simulink model "SWC_ETE_type"  (R2024a)
settings: Solver=FixedStepDiscrete  StartTime=0.0  StopTime=10.0  RelTol=1e-3
values from neighbouring files (symbols this model uses):
  C_FOC_SAMPLE_TIME = single(0.0001)    [vcu_local_hdr.m]
  ENUM_SENSORFOCMODE_CURRENTRDCTEMP = uint8(  2  )    [vcu_local_hdr.m]
  ENUM_SENSORFOCMODE_FAKERDC = uint8(  1  )    [vcu_local_hdr.m]
  ENUM_SENSORFOCMODE_RDCALIGN = uint8(  3  )    [vcu_local_hdr.m]
  ENUM_SENSORMODE_RDC = uint8(  0  )    [vcu_local_hdr.m]
  FALSE = boolean( 0 )    [vcu_local_hdr.m]
  MINUSONE_PI = single( -pi)    [vcu_local_hdr.m]
  PI = single( pi )    [vcu_local_hdr.m]
  SPD_GAIN = single(2*pi/60)    [vcu_local_hdr.m]
  TRUE = boolean( 1 )    [vcu_local_hdr.m]
  TWO_PI = single( 2*pi)    [vcu_local_hdr.m]
  ZERO_FLOAT = single(0)    [vcu_local_hdr.m]
undefined symbols (not defined in the file or in its folder): KFOC_25Amb_degC, KFOC_ADCReadEnum_enum, KFOC_DCBusLPF_c, KFOC_DCBusUseRaw_flg, KFOC_DCBusVoltage_V_ovrdflg, KFOC_DCBusVoltage_V_ovrdval, KFOC_FltActn_flg_ovrdflg, KFOC_FltActn_flg_ovrdfval, KFOC_GateICDisable_flg, KFOC_GateICEnable_flg, KFOC_GateICTempConst_raw, KFOC_IdCmd_A_ovrdflg, KFOC_IdCmd_A_ovrdfval, KFOC_IqCmd_A_ovrdflg, KFOC_IqCmd_A_ovrdfval, KFOC_OpMod_enum, KFOC_OpMod_enum_ovrdflg, KFOC_OpMod_enum_ovrdval, KFOC_PosnOffset_flg_ovrdflg, KFOC_PosnOffset_rad_ovrdval, KFOC_PWMidle_flg, KFOC_RotPosnOffset_rad_ovrdflg, KFOC_RotPosnOffset_rad_ovrdval, KFOC_SensorMode_enum, KFOC_SpdCmd_RPM, KFOC_TCTS_const, KFOC_VdCmd_V, KFOC_VqCmd_V, KFOC_VTS25_V
libraries: simulink x6, rot x2, GRC_Lib x1, pcs_grc x1, rot_grc x1, hdlsllib x1, CCM_FVT x1, dgh_grc x1, pdc_grc x1
(part 2 of 2)

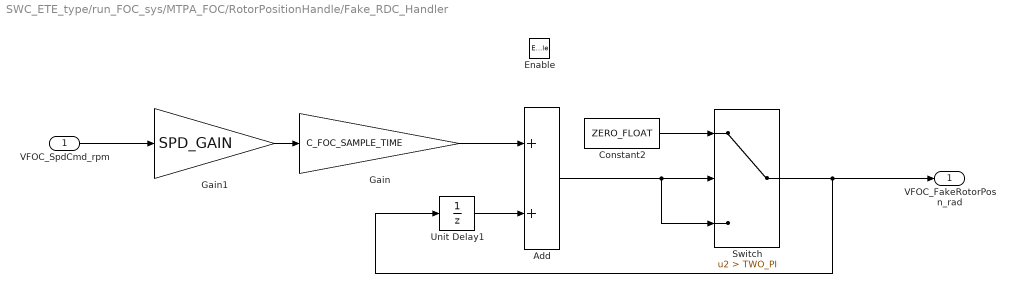
== system SWC_ETE_type/run_FOC_sys/MTPA_FOC/RotorPositionHandle/Fake_RDC_Handler ==
  VFOC_SpdCmd_rpm : Inport
  Enable : EnablePort
  Add : Sum
  Constant2 : Constant  Value=ZERO_FLOAT
  Gain : Gain  Gain=C_FOC_SAMPLE_TIME
  Gain1 : Gain  Gain=SPD_GAIN
  Switch : Switch  Criteria=u2 > Threshold  Threshold=TWO_PI  SaturateOnIntegerOverflow=off  InputSameDT=off
      settings: AttributesFormatString=%<Criteria>
  Unit Delay1 : UnitDelay  SampleTime=-1  HasFrameUpgradeWarning=on
  VFOC_FakeRotorPosn_rad : Outport
  wires:
  Add/1 -> Switch/3, Switch/2
  VFOC_SpdCmd_rpm/1 -> Gain1/1
  Gain1/1 -> Gain/1
  Unit Delay1/1 -> Add/2
  Switch/1 -> VFOC_FakeRotorPosn_rad/1, Unit Delay1/1
  Gain/1 -> Add/1
  Constant2/1 -> Switch/1

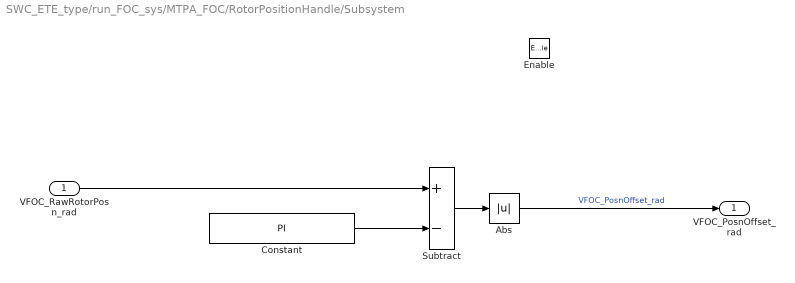
== system SWC_ETE_type/run_FOC_sys/MTPA_FOC/RotorPositionHandle/Subsystem ==
  VFOC_RawRotorPosn_rad : Inport
  Enable : EnablePort
  Abs : Abs  SaturateOnIntegerOverflow=off
  Constant : Constant  Value=PI
  Subtract : Sum  Inputs=+-
  VFOC_PosnOffset_rad : Outport
  wires:
  VFOC_RawRotorPosn_rad/1 -> Subtract/1
  Subtract/1 -> Abs/1
  Constant/1 -> Subtract/2
  Abs/1 -> VFOC_PosnOffset_rad/1  "VFOC_PosnOffset_rad"
